simulink model "model"  (Simulink 7.5)
settings: Solver=ode45  StartTime=0.0  StopTime=20.0  RelTol=1e-3
settings Model: Creator=168092  LastModifiedBy=TC

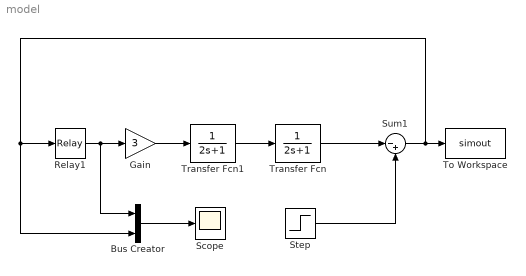
== system model ==
  Bus Creator : BusCreator  Inputs=2
  Gain : Gain  Gain=3  ParameterDataType=fixdt(1, 16)  ParameterScaling=2^0  OutDataType=fixdt(1, 16)  OutScaling=2^0
  Relay1 : Relay  OutDataType=fixdt(1, 16)  OutScaling=2^0
  Scope : Scope
  Step : Step  Time=0  After=2  SampleTime=0
  Sum1 : Sum  Inputs=|-+  OutDataType=fixdt(1, 16)  OutScaling=2^0
  To Workspace : ToWorkspace  VariableName=simout  SampleTime=-1  SaveFormat=Structure
  Transfer Fcn : TransferFcn  Denominator=[2 1]
  Transfer Fcn1 : TransferFcn  Denominator=[2 1]
  wires:
  Step/1 -> Sum1/2
  Transfer Fcn/1 -> Sum1/1
  Sum1/1 -> To Workspace/1, Bus Creator/2, Relay1/1
  Relay1/1 -> Gain/1, Bus Creator/1
  Gain/1 -> Transfer Fcn1/1
  Transfer Fcn1/1 -> Transfer Fcn/1
  Bus Creator/1 -> Scope/1
